simulink model "HH"  (Simulink 10.1)
settings: Solver=ode1  StartTime=0.0  StopTime=200  FixedStep=0.001  RelTol=1e-3  EnableMultiTasking=on
values from neighbouring files (symbols this model uses):
  EK = -12    [HHparameters.m]
  EL = 10.613    [HHparameters.m]
  ENa = 115    [HHparameters.m]
  gK = 36    [HHparameters.m]
  gL = 0.3    [HHparameters.m]
  gNa = 120    [HHparameters.m]
  h0 = 1    [HHparameters.m]
  m0 = 0    [HHparameters.m]
  n0 = 0    [HHparameters.m]
  V0 = 0    [HHparameters.m]
settings Model: Creator=MURAT  LastModifiedBy=Andreas
settings DataIOCC: LimitDataPoints=on  SignalLoggingSaveFormat=ModelDataLogs
settings OptimizationCC: InitFltsAndDblsToZero=on
settings DebuggingCC: SaveWithParameterizedLinksMsg=none  SignalResolutionControl=TryResolveAllWithWarning  SolverPrmCheckMsg=warning  FcnCallInpInsideContextMsg=warning
settings SFSimCC: SimUseLocalCustomCode=on  CustomCodeUndefinedFunction=FilterOut
settings RTWCC: RTWUseLocalCustomCode=on
settings GRTTargetCC: TargetFcnLib=ansi_tfl_tmw.mat
settings ConfigComp: CovExternalEMLEnable=on

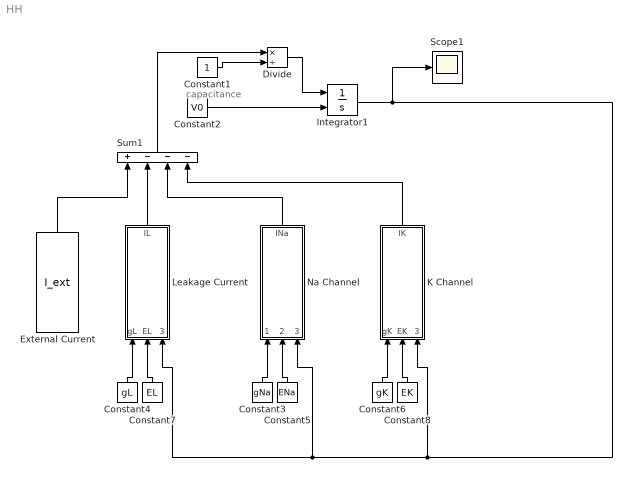
== system HH ==
  note: capacitance
  Constant1 : Constant
  Constant2 : Constant  Value=V0
  Constant3 : Constant  Value=gNa
  Constant4 : Constant  Value=gL
  Constant5 : Constant  Value=ENa
  Constant6 : Constant  Value=gK
  Constant7 : Constant  Value=EL
  Constant8 : Constant  Value=EK
  Divide : Product  Inputs=*/
  External Current : FromWorkspace  VariableName=I_ext
  Integrator1 : Integrator  InitialConditionSource=external
  K Channel : Subsystem
  Leakage Current : Subsystem
  Na Channel : Subsystem
  Scope1 : Scope
  Sum1 : Sum  Inputs=+---
  wires:
  Leakage Current/1(IL) -> Sum1/2
  Na Channel/1(INa) -> Sum1/3
  K Channel/1(IK) -> Sum1/4
  External Current/1 -> Sum1/1
  Constant2/1 -> Integrator1/2
  Constant3/1 -> Na Channel/1(gNa)
  Constant6/1 -> K Channel/1(gK)
  Constant4/1 -> Leakage Current/1(gL)
  Constant7/1 -> Leakage Current/2(EL)
  Constant5/1 -> Na Channel/2(ENa)
  Constant8/1 -> K Channel/2(EK)
  Integrator1/1 -> Scope1/1, Leakage Current/3(Vm), Na Channel/3(Vm), K Channel/3(Vm)
  Sum1/1 -> Divide/1
  Divide/1 -> Integrator1/1
  Constant1/1 -> Divide/2

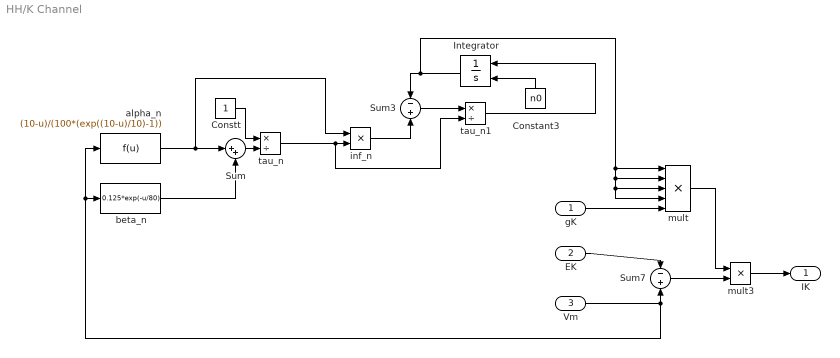
== system HH/K Channel ==
  gK : Inport
  EK : Inport  Port=2
  Vm : Inport  Port=3
  Constant3 : Constant  Value=n0
  Constt : Constant
  Integrator : Integrator  InitialConditionSource=external
  Sum : Sum  Inputs=|++
  Sum3 : Sum  Inputs=-+
  Sum7 : Sum  Inputs=-+
  alpha_n : Fcn  Expr=(10-u)/(100*(exp((10-u)/10)-1))
  beta_n : Fcn  Expr=0.125*exp(-u/80)
  inf_n : Product  Inputs=**
  mult : Product  Inputs=*****
  mult3 : Product  Inputs=**
  tau_n : Product  Inputs=*/
  tau_n1 : Product  Inputs=*/
  IK : Outport
  wires:
  mult3/1 -> IK/1
  Vm/1 -> Sum7/2, beta_n/1, alpha_n/1
  EK/1 -> Sum7/1
  gK/1 -> mult/5
  Sum7/1 -> mult3/2
  mult/1 -> mult3/1
  Constant3/1 -> Integrator/2
  tau_n1/1 -> Integrator/1
  Sum3/1 -> tau_n1/1
  inf_n/1 -> Sum3/2
  Integrator/1 -> Sum3/1, mult/1, mult/2, mult/3, mult/4
  tau_n/1 -> inf_n/2, tau_n1/2
  Sum/1 -> tau_n/2
  Constt/1 -> tau_n/1
  beta_n/1 -> Sum/2
  alpha_n/1 -> Sum/1, inf_n/1

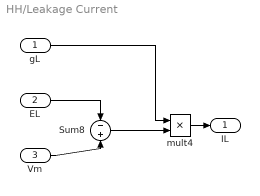
== system HH/Leakage Current ==
  gL : Inport
  EL : Inport  Port=2
  Vm : Inport  Port=3
  Sum8 : Sum  Inputs=-+
  mult4 : Product  Inputs=**
  IL : Outport
  wires:
  Sum8/1 -> mult4/2
  gL/1 -> mult4/1
  EL/1 -> Sum8/1
  Vm/1 -> Sum8/2
  mult4/1 -> IL/1

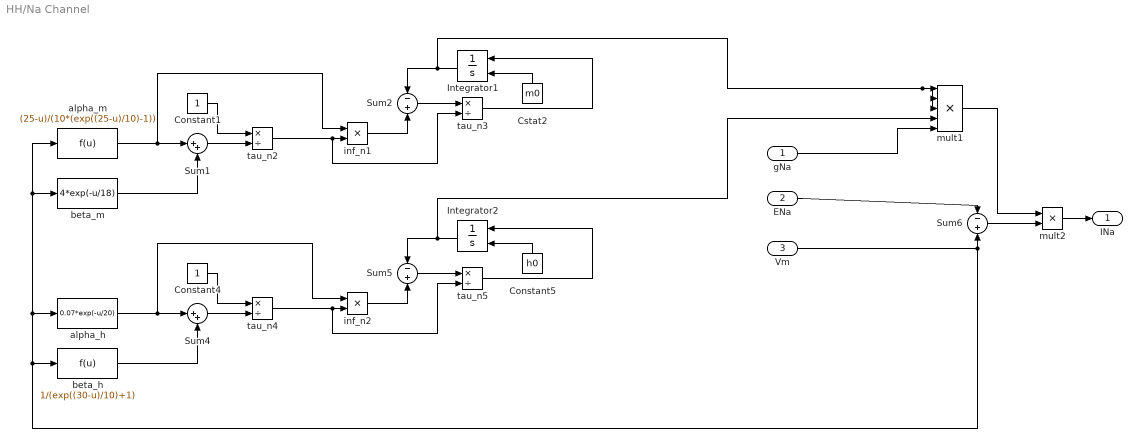
== system HH/Na Channel ==
  gNa : Inport
  ENa : Inport  Port=2
  Vm : Inport  Port=3
  Constant1 : Constant
  Constant4 : Constant
  Constant5 : Constant  Value=h0
  Cstat2 : Constant  Value=m0
  Integrator1 : Integrator  InitialConditionSource=external
  Integrator2 : Integrator  InitialConditionSource=external
  Sum1 : Sum  Inputs=|++
  Sum2 : Sum  Inputs=-+
  Sum4 : Sum  Inputs=|++
  Sum5 : Sum  Inputs=-+
  Sum6 : Sum  Inputs=-+
  alpha_h : Fcn  Expr=0.07*exp(-u/20)
  alpha_m : Fcn  Expr=(25-u)/(10*(exp((25-u)/10)-1))
  beta_h : Fcn  Expr=1/(exp((30-u)/10)+1)
  beta_m : Fcn  Expr=4*exp(-u/18)
  inf_n1 : Product  Inputs=**
  inf_n2 : Product  Inputs=**
  mult1 : Product  Inputs=*****
  mult2 : Product  Inputs=**
  tau_n{2..5} (4 alike) : Product  Inputs=*/
  INa : Outport
  wires:
  alpha_m/1 -> Sum1/1, inf_n1/1
  beta_m/1 -> Sum1/2
  Constant1/1 -> tau_n2/1
  Sum1/1 -> tau_n2/2
  alpha_h/1 -> Sum4/1, inf_n2/1
  beta_h/1 -> Sum4/2
  Constant4/1 -> tau_n4/1
  Sum4/1 -> tau_n4/2
  tau_n2/1 -> inf_n1/2, tau_n3/2
  Integrator1/1 -> Sum2/1, mult1/2, mult1/3, mult1/1
  inf_n1/1 -> Sum2/2
  Sum2/1 -> tau_n3/1
  tau_n4/1 -> inf_n2/2, tau_n5/2
  Integrator2/1 -> Sum5/1, mult1/4
  inf_n2/1 -> Sum5/2
  Sum5/1 -> tau_n5/1
  tau_n5/1 -> Integrator2/1
  Constant5/1 -> Integrator2/2
  tau_n3/1 -> Integrator1/1
  Cstat2/1 -> Integrator1/2
  Sum6/1 -> mult2/2
  gNa/1 -> mult1/5
  mult1/1 -> mult2/1
  ENa/1 -> Sum6/1
  Vm/1 -> Sum6/2, alpha_m/1, beta_m/1, alpha_h/1, beta_h/1
  mult2/1 -> INa/1
